simulink model "StandardModel_tl"  (Simulink 7.5)
settings: Solver=FixedStepDiscrete  StartTime=0.0  StopTime=10.0  FixedStep=0.01  RelTol=1e-3
PreLoadFcn:
  | if exist('tl_preloadfcn','file'), tl_preloadfcn(gcs,101); end
PostLoadFcn:
  | if exist('tl_postloadfcn','file'), tl_postloadfcn(gcs,101); end
InitFcn:
  | if exist('tlds_init','file'), tlds_init(gcs); end
StartFcn:
  | if exist('tlds_start','file'), tlds_start(gcs); end
StopFcn:
  | if exist('tlds_stop','file'), tlds_stop(gcs); end
libraries: tllib x6
PreSaveFcn:
  | if exist('tl_presavefcn','file'), tl_presavefcn(gcs); end
settings Model: DS_PROJECTFILE=StandardModel.dd  TL_MAIN_DATA={'codeopt',{'optlevel',0,'stateactcodinglimit',1},'logopt',{'plotinterval',0.1},'date',735991.67578921292,'advcodeopt',{'ExtendedBlockComments';'on';'GenerateEmptyConditionalBranches';'on';'PolySpaceSupport';'on'}}  TLRevision=101  Creator=alex  LastModifiedBy=alex  BufferReuse=off
settings DataIOCC: SaveFormat=StructureWithTime
settings OptimizationCC: BlockReduction=off  OptimizeBlockIOStorage=off  BufferReuse=off  ExpressionFolding=off  LocalBlockOutputs=off  InitFltsAndDblsToZero=on
settings DebuggingCC: SaveWithParameterizedLinksMsg=none  SignalResolutionControl=TryResolveAllWithWarning  MultiTaskDSMMsg=warning  MultiTaskCondExecSysMsg=none
settings RTWCC: IncludeERTFirstTime=on
settings GRTTargetCC: TargetFcnLib=ansi_tfl_tmw.mat

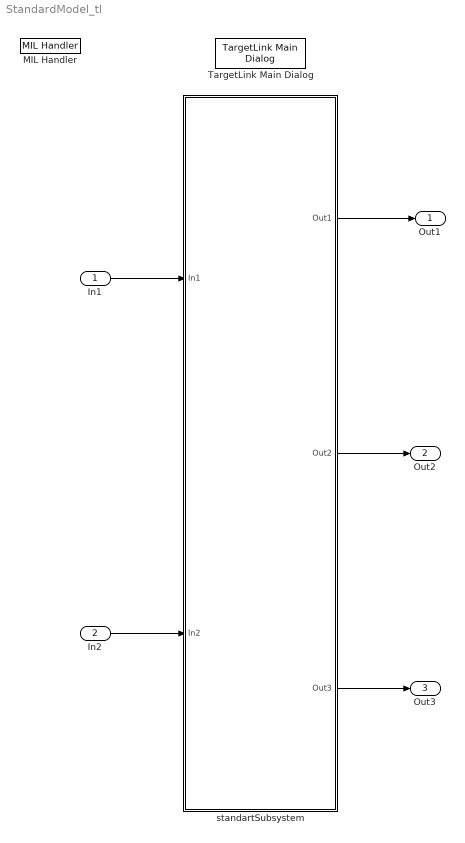
== system StandardModel_tl ==
  In1 : Inport  OutDataType=sfix(16)  OutScaling=2^0
  In2 : Inport  Port=2  OutDataType=sfix(16)  OutScaling=2^0
  MIL Handler : tllib/MIL Handler  data={'date',735991.67578725691}
  TargetLink Main Dialog : tllib/TargetLink Main Dialog  SystemSampleTime=-1
  standartSubsystem : Subsystem  Tag=TargetLink Simulation Frame
      settings: CopyFcn=if exist('tl_copyfcn','file'), tl_copyfcn(gcbh); end  NameChangeFcn=if exist('tl_framenamechangefcn','file'), tl_framenamechangefcn(gcbh); end
      settings: OpenFcn=|
      | if exist('open_tlsubsystem','file')
      |    open_tlsubsystem(gcbh);
      | else
      |    tlsubsystem = ...
      |       find_system(gcb, ...
      |       'LookUnderMasks','on', ...
      |       'FollowLinks','on', ...
      |       'Tag','MIL Subsystem');
      |    open_system(tlsubsystem);
      | end
      mask Type: TL_SimFrame
      mask Display: disp('TargetLink\nModel-\nin-the-loop\nmode')
  Out1 : Outport  OutDataType=sfix(16)  OutScaling=2^0
  Out2 : Outport  Port=2  OutDataType=sfix(16)  OutScaling=2^0
  Out3 : Outport  Port=3  OutDataType=sfix(16)  OutScaling=2^0
  wires:
  In1/1 -> standartSubsystem/1(In1)
  In2/1 -> standartSubsystem/2(In2)
  standartSubsystem/1(Out1) -> Out1/1
  standartSubsystem/2(Out2) -> Out2/1
  standartSubsystem/3(Out3) -> Out3/1

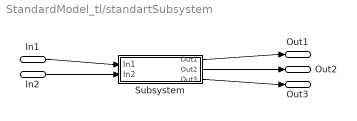
== system StandardModel_tl/standartSubsystem ==
  In1 : Inport  OutDataType=sfix(16)  OutScaling=2^0
  In2 : Inport  Port=2  OutDataType=sfix(16)  OutScaling=2^0
  Subsystem : Subsystem
      settings: OpenFcn=warndlg(get_param(gcb,'MaskHelp'),'Serious Warning');
      mask Type: TL_Enable
      mask Help: This subsystem keeps the TargetLink subsystem (subsystem with TargetLink blocks for production code generation), and is needed for the TargetLink simulation frame to work properly. DO NOT DELETE OR MODIFY IT!
  Out1 : Outport  OutDataType=sfix(16)  OutScaling=2^0
  Out2 : Outport  Port=2  OutDataType=sfix(16)  OutScaling=2^0
  Out3 : Outport  Port=3  OutDataType=sfix(16)  OutScaling=2^0
  wires:
  In1/1 -> Subsystem/1(In1)
  In2/1 -> Subsystem/2(In2)
  Subsystem/1(Out1) -> Out1/1
  Subsystem/2(Out2) -> Out2/1
  Subsystem/3(Out3) -> Out3/1

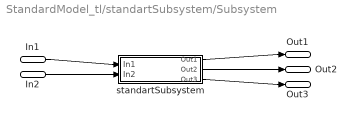
== system StandardModel_tl/standartSubsystem/Subsystem ==
  In1 : Inport  OutDataType=sfix(16)  OutScaling=2^0
  In2 : Inport  Port=2  OutDataType=sfix(16)  OutScaling=2^0
  standartSubsystem : Subsystem  Tag=MIL Subsystem  Description=a
      settings: CopyFcn=if exist('tl_copyfcn','file'), tl_copyfcn(gcbh); end  NameChangeFcn=if exist('tl_namechangefcn','file'), tl_namechangefcn(gcbh); end  DestroyFcn=if exist('update_tl_main_dlg','file'), update_tl_main_dlg('TL_subs_display'); end
      mask Display: disp('TargetLink Subsystem')
  Out1 : Outport  OutDataType=sfix(16)  OutScaling=2^0
  Out2 : Outport  Port=2  OutDataType=sfix(16)  OutScaling=2^0
  Out3 : Outport  Port=3  OutDataType=sfix(16)  OutScaling=2^0
  wires:
  In1/1 -> standartSubsystem/1(In1)
  In2/1 -> standartSubsystem/2(In2)
  standartSubsystem/1(Out1) -> Out1/1
  standartSubsystem/2(Out2) -> Out2/1
  standartSubsystem/3(Out3) -> Out3/1

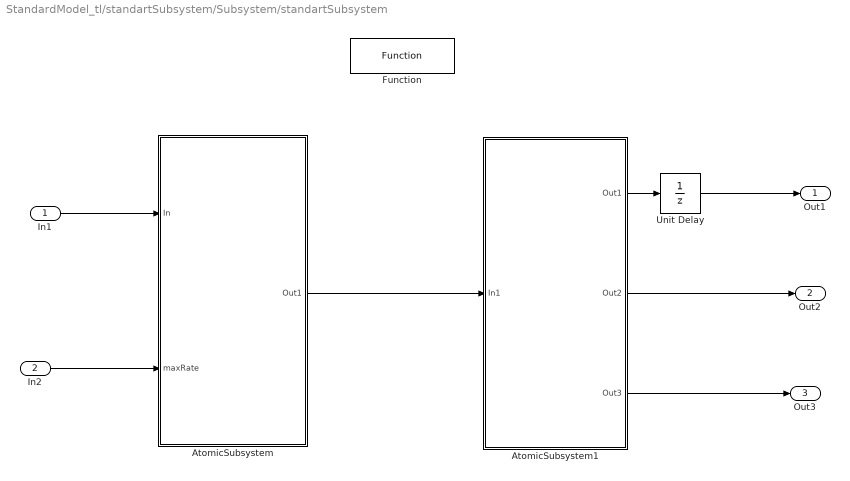
== system StandardModel_tl/standartSubsystem/Subsystem/standartSubsystem ==
  In1 : Inport  PortDimensions=1  OutDataType=sfix(16)  OutScaling=2^0  mask(TL_Inport){data={'logdata',{'plotchannels',[]},'date',735991.6757871412}}
      settings: DeleteFcn=if exist('delete_tlblock','file')==2,delete_tlblock(gcbh);end  OpenFcn=if exist('tl_open_blockdlg','file')==2,tl_open_blockdlg(gcbh);else,open_system(gcbh,'parameter');end
      settings: CopyFcn=|
      | if exist('tl_reset_reviewflag','file')==2
      |     tl_reset_reviewflag(gcbh);
      | end
      | if exist('tl_check_ports','file')
      |     tl_check_ports(gcbh);
      | end
      settings: NameChangeFcn=|
      | if exist('rename_tlblock','file')==2,rename_tlblock(gcbh);end
      | if exist('tl_check_ports','file'), tl_check_ports(gcbh); end
      mask Help: eval(['if exist(''tl_online_help'',''file'') == 2, tl_online_help(''Topic'',''TL_Inport''),else, web([''jar:file:///'',matlabroot,''/help/toolbox/simulink/help.jar!/slref/' lower(get_param(gcbh,'Blocktype')) '.html''], ''-helpbrowser''),end'])
      mask Display: plot([0.2 0.35 NaN 0.65 0.8],[0 1 NaN 0 1]);
  In2 : Inport  Port=2  PortDimensions=1  OutDataType=sfix(16)  OutScaling=2^0  mask(TL_Inport){data={'logdata',{'plotchannels',[]},'output',{'max',300,'min',-800,'lsb',2^-2,'offset',-4},'date',735991.67578673607}}
      settings: DeleteFcn=if exist('delete_tlblock','file')==2,delete_tlblock(gcbh);end  OpenFcn=if exist('tl_open_blockdlg','file')==2,tl_open_blockdlg(gcbh);else,open_system(gcbh,'parameter');end
      settings: CopyFcn=|
      | if exist('tl_reset_reviewflag','file')==2
      |     tl_reset_reviewflag(gcbh);
      | end
      | if exist('tl_check_ports','file')
      |     tl_check_ports(gcbh);
      | end
      settings: NameChangeFcn=|
      | if exist('rename_tlblock','file')==2,rename_tlblock(gcbh);end
      | if exist('tl_check_ports','file'), tl_check_ports(gcbh); end
      mask Help: eval(['if exist(''tl_online_help'',''file'') == 2, tl_online_help(''Topic'',''TL_Inport''),else, web([''jar:file:///'',matlabroot,''/help/toolbox/simulink/help.jar!/slref/' lower(get_param(gcbh,'Blocktype')) '.html''], ''-helpbrowser''),end'])
      mask Display: plot([0.2 0.35 NaN 0.65 0.8],[0 1 NaN 0 1]);
  AtomicSubsystem : Subsystem  TreatAsAtomicUnit=on
  AtomicSubsystem1 : Subsystem  TreatAsAtomicUnit=on
  Function : tllib/Function  SystemSampleTime=-1  data={'date',735991.67578028934}
  Unit Delay : UnitDelay  X0=-2  SampleTime=-1  mask(TL_UnitDelay){data={'logdata',{'plotchannels',[]},'date',735991.6757827315}}
      settings: CopyFcn=set_param(gcb,'ReferenceBlock',''); set_param(gcb,'Tag','COPIED_DURING_UPGRADE');set_param(gcb,'CopyFcn','');  DeleteFcn=if exist('delete_tlblock','file')==2,delete_tlblock(gcbh);end  NameChangeFcn=if exist('rename_tlblock','file')==2,rename_tlblock(gcbh);end  OpenFcn=if exist('tl_open_blockdlg','file')==2,tl_open_blockdlg(gcbh);else,open_system(gcbh,'parameter');end
      mask Help: eval(['if exist(''tl_online_help'',''file'') == 2, tl_online_help(''Topic'',''TL_UnitDelay''),else, web([''jar:file:///'',matlabroot,''/help/toolbox/simulink/help.jar!/slref/' lower(get_param(gcbh,'Blocktype')) '.html''], ''-helpbrowser''),end'])
      mask Display: plot([-0.05, 1.05, NaN, -0.05, 1.05],[.01, .01, NaN, .99, .99])
  Out1 : Outport  PortDimensions=1  OutDataType=sfix(16)  OutScaling=2^0  mask(TL_Outport){data={'logdata',{'plotchannels',[]},'output',{'lsb',2^-1,'offset',-3,'checkmin',1,'checkmax',1},'date',735991.6757824074}}
      settings: DeleteFcn=if exist('delete_tlblock','file')==2,delete_tlblock(gcbh);end  OpenFcn=if exist('tl_open_blockdlg','file')==2,tl_open_blockdlg(gcbh);else,open_system(gcbh,'parameter');end
      settings: CopyFcn=|
      | if exist('tl_reset_reviewflag','file')==2
      |     tl_reset_reviewflag(gcbh);
      | end
      | if exist('tl_check_ports','file')
      |     tl_check_ports(gcbh);
      | end
      settings: NameChangeFcn=|
      | if exist('rename_tlblock','file')==2,rename_tlblock(gcbh);end
      | if exist('tl_check_ports','file'), tl_check_ports(gcbh); end
      mask Help: eval(['if exist(''tl_online_help'',''file'') == 2, tl_online_help(''Topic'',''TL_Outport''),else, web([''jar:file:///'',matlabroot,''/help/toolbox/simulink/help.jar!/slref/' lower(get_param(gcbh,'Blocktype')) '.html''], ''-helpbrowser''),end'])
      mask Display: plot([0.2 0.35 NaN 0.65 0.8],[0 1 NaN 0 1]);
  Out2 : Outport  Port=2  PortDimensions=1  OutDataType=sfix(16)  OutScaling=2^0  mask(TL_Outport){data={'logdata',{'plotchannels',[]},'date',735991.67578196758}}
      settings: DeleteFcn=if exist('delete_tlblock','file')==2,delete_tlblock(gcbh);end  OpenFcn=if exist('tl_open_blockdlg','file')==2,tl_open_blockdlg(gcbh);else,open_system(gcbh,'parameter');end
      settings: CopyFcn=|
      | if exist('tl_reset_reviewflag','file')==2
      |     tl_reset_reviewflag(gcbh);
      | end
      | if exist('tl_check_ports','file')
      |     tl_check_ports(gcbh);
      | end
      settings: NameChangeFcn=|
      | if exist('rename_tlblock','file')==2,rename_tlblock(gcbh);end
      | if exist('tl_check_ports','file'), tl_check_ports(gcbh); end
      mask Help: eval(['if exist(''tl_online_help'',''file'') == 2, tl_online_help(''Topic'',''TL_Outport''),else, web([''jar:file:///'',matlabroot,''/help/toolbox/simulink/help.jar!/slref/' lower(get_param(gcbh,'Blocktype')) '.html''], ''-helpbrowser''),end'])
      mask Display: plot([0.2 0.35 NaN 0.65 0.8],[0 1 NaN 0 1]);
  Out3 : Outport  Port=3  PortDimensions=1  OutDataType=sfix(16)  OutScaling=2^0  mask(TL_Outport){data={'logdata',{'plotchannels',[]},'output',{'type','Int32'},'date',735991.67578146991}}
      settings: DeleteFcn=if exist('delete_tlblock','file')==2,delete_tlblock(gcbh);end  OpenFcn=if exist('tl_open_blockdlg','file')==2,tl_open_blockdlg(gcbh);else,open_system(gcbh,'parameter');end
      settings: CopyFcn=|
      | if exist('tl_reset_reviewflag','file')==2
      |     tl_reset_reviewflag(gcbh);
      | end
      | if exist('tl_check_ports','file')
      |     tl_check_ports(gcbh);
      | end
      settings: NameChangeFcn=|
      | if exist('rename_tlblock','file')==2,rename_tlblock(gcbh);end
      | if exist('tl_check_ports','file'), tl_check_ports(gcbh); end
      mask Help: eval(['if exist(''tl_online_help'',''file'') == 2, tl_online_help(''Topic'',''TL_Outport''),else, web([''jar:file:///'',matlabroot,''/help/toolbox/simulink/help.jar!/slref/' lower(get_param(gcbh,'Blocktype')) '.html''], ''-helpbrowser''),end'])
      mask Display: plot([0.2 0.35 NaN 0.65 0.8],[0 1 NaN 0 1]);
  wires:
  AtomicSubsystem1/3(Out3) -> Out3/1
  AtomicSubsystem1/2(Out2) -> Out2/1
  Unit Delay/1 -> Out1/1
  In2/1 -> AtomicSubsystem/2(maxRate)
  In1/1 -> AtomicSubsystem/1(In)
  AtomicSubsystem/1(Out1) -> AtomicSubsystem1/1(In1)
  AtomicSubsystem1/1(Out1) -> Unit Delay/1

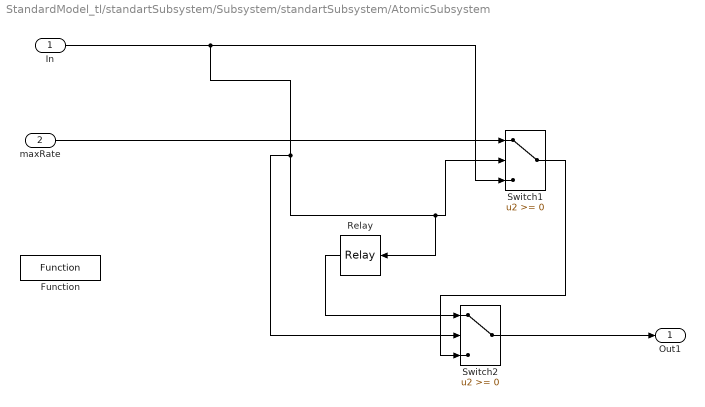
== system StandardModel_tl/standartSubsystem/Subsystem/standartSubsystem/AtomicSubsystem ==
  In : Inport  PortDimensions=1  OutDataType=sfix(16)  OutScaling=2^0  mask(TL_Inport){data={'logdata',{'plotchannels',[]},'output',{'class','FCN_ARG'},'date',735991.67578631942}}
      settings: CopyFcn=if exist('tl_reset_reviewflag','file')==2,tl_reset_reviewflag(gcbh);end  DeleteFcn=if exist('delete_tlblock','file')==2,delete_tlblock(gcbh);end  NameChangeFcn=if exist('rename_tlblock','file')==2,rename_tlblock(gcbh);end  OpenFcn=if exist('tl_open_blockdlg','file')==2,tl_open_blockdlg(gcbh);else,open_system(gcbh,'parameter');end
      mask Help: eval(['if exist(''tl_online_help'',''file'') == 2, tl_online_help(''Topic'',''TL_Inport''),else, web([''jar:file:///'',matlabroot,''/help/toolbox/simulink/help.jar!/slref/' lower(get_param(gcbh,'Blocktype')) '.html''], ''-helpbrowser''),end'])
      mask Display: plot([0.2 0.35 NaN 0.65 0.8],[0 1 NaN 0 1]);
  maxRate : Inport  Port=2  PortDimensions=1  OutDataType=sfix(16)  OutScaling=2^0  mask(TL_Inport){data={'logdata',{'plotchannels',[]},'output',{'class','FCN_REF_ARG'},'date',735991.6757859143}}
      settings: CopyFcn=if exist('tl_reset_reviewflag','file')==2,tl_reset_reviewflag(gcbh);end  DeleteFcn=if exist('delete_tlblock','file')==2,delete_tlblock(gcbh);end  NameChangeFcn=if exist('rename_tlblock','file')==2,rename_tlblock(gcbh);end  OpenFcn=if exist('tl_open_blockdlg','file')==2,tl_open_blockdlg(gcbh);else,open_system(gcbh,'parameter');end
      mask Help: eval(['if exist(''tl_online_help'',''file'') == 2, tl_online_help(''Topic'',''TL_Inport''),else, web([''jar:file:///'',matlabroot,''/help/toolbox/simulink/help.jar!/slref/' lower(get_param(gcbh,'Blocktype')) '.html''], ''-helpbrowser''),end'])
      mask Display: plot([0.2 0.35 NaN 0.65 0.8],[0 1 NaN 0 1]);
  Function : tllib/Function  SystemSampleTime=-1  data={'stepfunctionclass','STATIC_FCN','date',735991.6757809954}
  Relay : Relay  OnSwitchValue=1  OffSwitchValue=-1  OutDataType=sfix(16)  OutScaling=2^0  mask(TL_Relay){data={'logdata',{'plotchannels',[]},'onoutput',{'class','CAL'},'offoutput',{'class','CAL'},'onswitch',{'class','CAL'},'offswitch',{'class','CAL'},'date',735991.67578543979}}
      settings: CopyFcn=set_param(gcb,'ReferenceBlock',''); set_param(gcb,'Tag','COPIED_DURING_UPGRADE');set_param(gcb,'CopyFcn','');  DeleteFcn=if exist('delete_tlblock','file')==2,delete_tlblock(gcbh);end  NameChangeFcn=if exist('rename_tlblock','file')==2,rename_tlblock(gcbh);end  OpenFcn=if exist('tl_open_blockdlg','file')==2,tl_open_blockdlg(gcbh);else,open_system(gcbh,'parameter');end
      mask Help: eval(['if exist(''tl_online_help'',''file'') == 2, tl_online_help(''Topic'',''TL_Relay''),else, web([''jar:file:///'',matlabroot,''/help/toolbox/simulink/help.jar!/slref/' lower(get_param(gcbh,'Blocktype')) '.html''], ''-helpbrowser''),end'])
      mask Display: plot([-0.05, 1.05, NaN, -0.05, 1.05],[.01, .01, NaN, .99, .99])
  Switch1 : Switch  OutDataType=sfix(16)  OutScaling=2^0  SaturateOnIntegerOverflow=on  InputSameDT=on  mask(TL_Switch){data={'logdata',{'plotchannels',[]},'threshold',{'class','CAL'},'date',735991.67578491895}}
      settings: CopyFcn=set_param(gcb,'ReferenceBlock',''); set_param(gcb,'Tag','COPIED_DURING_UPGRADE');set_param(gcb,'CopyFcn','');  DeleteFcn=if exist('delete_tlblock','file')==2,delete_tlblock(gcbh);end  NameChangeFcn=if exist('rename_tlblock','file')==2,rename_tlblock(gcbh);end  OpenFcn=if exist('tl_open_blockdlg','file')==2,tl_open_blockdlg(gcbh);else,open_system(gcbh,'parameter');end
      mask Help: eval(['if exist(''tl_online_help'',''file'') == 2, tl_online_help(''Topic'',''TL_Switch''),else, web([''jar:file:///'',matlabroot,''/help/toolbox/simulink/help.jar!/slref/' lower(get_param(gcbh,'Blocktype')) '.html''], ''-helpbrowser''),end'])
      mask Display: plot([-0.05, 1.05, NaN, -0.05, 1.05],[.01, .01, NaN, .99, .99])
  Switch2 : Switch  OutDataType=sfix(16)  OutScaling=2^0  SaturateOnIntegerOverflow=on  InputSameDT=on  mask(TL_Switch){data={'logdata',{'plotchannels',[]},'threshold',{'class','CAL'},'date',735991.67578460649}}
      settings: CopyFcn=set_param(gcb,'ReferenceBlock',''); set_param(gcb,'Tag','COPIED_DURING_UPGRADE');set_param(gcb,'CopyFcn','');  DeleteFcn=if exist('delete_tlblock','file')==2,delete_tlblock(gcbh);end  NameChangeFcn=if exist('rename_tlblock','file')==2,rename_tlblock(gcbh);end  OpenFcn=if exist('tl_open_blockdlg','file')==2,tl_open_blockdlg(gcbh);else,open_system(gcbh,'parameter');end
      mask Help: eval(['if exist(''tl_online_help'',''file'') == 2, tl_online_help(''Topic'',''TL_Switch''),else, web([''jar:file:///'',matlabroot,''/help/toolbox/simulink/help.jar!/slref/' lower(get_param(gcbh,'Blocktype')) '.html''], ''-helpbrowser''),end'])
      mask Display: plot([-0.05, 1.05, NaN, -0.05, 1.05],[.01, .01, NaN, .99, .99])
  Out1 : Outport  PortDimensions=1  OutDataType=sfix(16)  OutScaling=2^0  mask(TL_Outport){data={'logdata',{'plotchannels',[]},'output',{'class','FCN_RETURN'},'date',735991.67578423605}}
      settings: CopyFcn=if exist('tl_reset_reviewflag','file')==2,tl_reset_reviewflag(gcbh);end  DeleteFcn=if exist('delete_tlblock','file')==2,delete_tlblock(gcbh);end  NameChangeFcn=if exist('rename_tlblock','file')==2,rename_tlblock(gcbh);end  OpenFcn=if exist('tl_open_blockdlg','file')==2,tl_open_blockdlg(gcbh);else,open_system(gcbh,'parameter');end
      mask Help: eval(['if exist(''tl_online_help'',''file'') == 2, tl_online_help(''Topic'',''TL_Outport''),else, web([''jar:file:///'',matlabroot,''/help/toolbox/simulink/help.jar!/slref/' lower(get_param(gcbh,'Blocktype')) '.html''], ''-helpbrowser''),end'])
      mask Display: plot([0.2 0.35 NaN 0.65 0.8],[0 1 NaN 0 1]);
  wires:
  Relay/1 -> Switch2/1
  Switch1/1 -> Switch2/3
  Switch2/1 -> Out1/1
  maxRate/1 -> Switch1/1
  In/1 -> Switch1/3, Switch1/2, Relay/1, Switch2/2

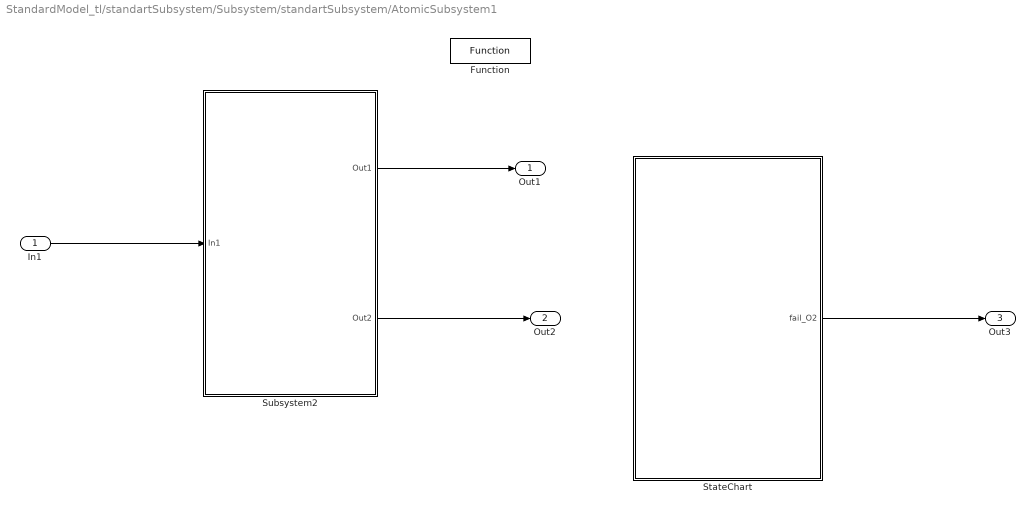
== system StandardModel_tl/standartSubsystem/Subsystem/standartSubsystem/AtomicSubsystem1 ==
  In1 : Inport  OutDataType=sfix(16)  OutScaling=2^0
  Function : tllib/Function  SystemSampleTime=-1  data={'date',735991.67578077549}
  StateChart : Stateflow chart  Description=Stateflow diagram to determine control system operating mode  TreatAsAtomicUnit=on
  Subsystem2 : Subsystem  TreatAsAtomicUnit=on
  Out1 : Outport  OutDataType=sfix(16)  OutScaling=2^0
  Out2 : Outport  Port=2  OutDataType=sfix(16)  OutScaling=2^0
  Out3 : Outport  Port=3  OutDataType=sfix(16)  OutScaling=2^0
  wires:
  Subsystem2/2(Out2) -> Out2/1
  In1/1 -> Subsystem2/1(In1)
  Subsystem2/1(Out1) -> Out1/1
  StateChart/1(fail_O2) -> Out3/1

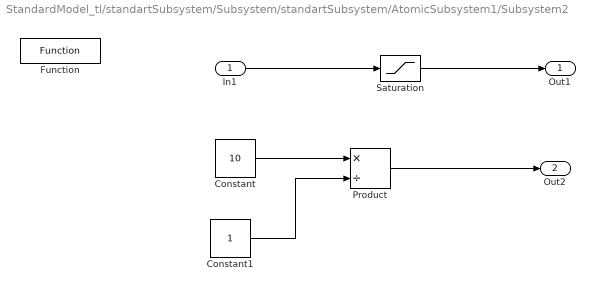
== system StandardModel_tl/standartSubsystem/Subsystem/standartSubsystem/AtomicSubsystem1/Subsystem2 ==
  In1 : Inport  OutDataType=sfix(16)  OutScaling=2^0
  Constant : Constant  Value=10  OutDataType=sfix(16)  OutScaling=2^0  mask(TL_Constant){data={'output',{'class','GLOBAL'},'date',735991.6757838194}}
      settings: CopyFcn=set_param(gcb,'ReferenceBlock',''); set_param(gcb,'Tag','COPIED_DURING_UPGRADE');set_param(gcb,'CopyFcn','');  DeleteFcn=if exist('delete_tlblock','file')==2,delete_tlblock(gcbh);end  NameChangeFcn=if exist('rename_tlblock','file')==2,rename_tlblock(gcbh);end  OpenFcn=if exist('tl_open_blockdlg','file')==2,tl_open_blockdlg(gcbh);else,open_system(gcbh,'parameter');end
      mask Help: eval(['if exist(''tl_online_help'',''file'') == 2, tl_online_help(''Topic'',''TL_Constant''),else, web([''jar:file:///'',matlabroot,''/help/toolbox/simulink/help.jar!/slref/' lower(get_param(gcbh,'Blocktype')) '.html''], ''-helpbrowser''),end'])
      mask Display: plot([-0.05, 1.05, NaN, -0.05, 1.05],[.01, .01, NaN, .99, .99])
  Constant1 : Constant  OutDataType=sfix(16)  OutScaling=2^0  mask(TL_Constant){data={'output',{'class','CAL'},'date',735991.67578361114}}
      settings: CopyFcn=set_param(gcb,'ReferenceBlock',''); set_param(gcb,'Tag','COPIED_DURING_UPGRADE');set_param(gcb,'CopyFcn','');  DeleteFcn=if exist('delete_tlblock','file')==2,delete_tlblock(gcbh);end  NameChangeFcn=if exist('rename_tlblock','file')==2,rename_tlblock(gcbh);end  OpenFcn=if exist('tl_open_blockdlg','file')==2,tl_open_blockdlg(gcbh);else,open_system(gcbh,'parameter');end
      mask Help: eval(['if exist(''tl_online_help'',''file'') == 2, tl_online_help(''Topic'',''TL_Constant''),else, web([''jar:file:///'',matlabroot,''/help/toolbox/simulink/help.jar!/slref/' lower(get_param(gcbh,'Blocktype')) '.html''], ''-helpbrowser''),end'])
      mask Display: plot([-0.05, 1.05, NaN, -0.05, 1.05],[.01, .01, NaN, .99, .99])
  Function : tllib/Function  SystemSampleTime=-1  data={'date',735991.67578054394}
  Product : Product  Inputs=*/  OutDataType=sfix(16)  OutScaling=2^0  RndMeth=Zero  mask(TL_Product){data={'logdata',{'plotchannels',[]},'date',735991.67578336806}}
      settings: CopyFcn=set_param(gcb,'ReferenceBlock',''); set_param(gcb,'Tag','COPIED_DURING_UPGRADE');set_param(gcb,'CopyFcn','');  DeleteFcn=if exist('delete_tlblock','file')==2,delete_tlblock(gcbh);end  NameChangeFcn=if exist('rename_tlblock','file')==2,rename_tlblock(gcbh);end  OpenFcn=if exist('tl_open_blockdlg','file')==2,tl_open_blockdlg(gcbh);else,open_system(gcbh,'parameter');end
      mask Help: eval(['if exist(''tl_online_help'',''file'') == 2, tl_online_help(''Topic'',''TL_Product''),else, web([''jar:file:///'',matlabroot,''/help/toolbox/simulink/help.jar!/slref/' lower(get_param(gcbh,'Blocktype')) '.html''], ''-helpbrowser''),end'])
      mask Display: plot([-0.05, 1.05, NaN, -0.05, 1.05],[.01, .01, NaN, .99, .99])
  Saturation : Saturate  UpperLimit=2  LowerLimit=0  OutDataType=sfix(16)  OutScaling=2^0  mask(TL_Saturate){data={'logdata',{'plotchannels',[]},'output',{'max',255,'min',0,'type','uint16'},'lowerlimit',{'class','CAL'},'upperlimit',{'class','CAL'},'date',735991.67578311346}}
      settings: CopyFcn=set_param(gcb,'ReferenceBlock',''); set_param(gcb,'Tag','COPIED_DURING_UPGRADE');set_param(gcb,'CopyFcn','');  DeleteFcn=if exist('delete_tlblock','file')==2,delete_tlblock(gcbh);end  NameChangeFcn=if exist('rename_tlblock','file')==2,rename_tlblock(gcbh);end  OpenFcn=if exist('tl_open_blockdlg','file')==2,tl_open_blockdlg(gcbh);else,open_system(gcbh,'parameter');end
      mask Help: eval(['if exist(''tl_online_help'',''file'') == 2, tl_online_help(''Topic'',''TL_Saturate''),else, web([''jar:file:///'',matlabroot,''/help/toolbox/simulink/help.jar!/slref/' lower(get_param(gcbh,'Blocktype')) '.html''], ''-helpbrowser''),end'])
      mask Display: plot([-0.05, 1.05, NaN, -0.05, 1.05],[.01, .01, NaN, .99, .99])
  Out1 : Outport  OutDataType=sfix(16)  OutScaling=2^0
  Out2 : Outport  Port=2  OutDataType=sfix(16)  OutScaling=2^0
  wires:
  In1/1 -> Saturation/1
  Saturation/1 -> Out1/1
  Constant1/1 -> Product/2
  Constant/1 -> Product/1
  Product/1 -> Out2/1

== stateflow chart standartSubsystem/Subsystem/standartSubsystem/AtomicSubsystem1/StateChart ==
  settings: updateMethod=DISCRETE  sampleTime=0.01  description=$TL$ functionname=$O; $TL$
  state OxygenSensMode [parallel]
    settings: executionOrder=1
    settings: description=|
        | This state determines the validity of the exhaust gas oxygen sensor (EGO) data.
        | $TL$ name=$C_X_$O$R; $TL$
    state O2_Normal
      entry: fail_O2 = 0;
      settings: description=|
          | Normal EGO sensor operation gives a reliable indication of excess oxygen in the exhaust gas, from which air/fuel mixture can be inferred.
          | $TL$ name=$C_X_$O$R; $TL$
    state O2_Fail
      entry: fail_O2 = 1;
      settings: description=|
          | The EGO sensor has failed.
          | $TL$ name=$C_X_$O$R; $TL$
    state O2_Warmup
      entry: fail_O2 = 1;
      settings: description=|
          | The EGO sensor must come up to temperature before its data is reliable.
          | $TL$ name=$C_X_$O$R; $TL$
    O2_Warmup -> O2_Normal : [Calvariable== 5]
      settings: description=It is assumed that the time o2_t_thresh is sufficient for the sensor to warm up to operational temperature.
    (default) -> O2_Warmup
    O2_Normal -> O2_Fail : [Calvariable == 7]
      settings: description=The failure condition is indicated by excessive output voltage.
  data: Calvariable parameter int32 [0..1] =1; fail_O2 output int32 [0..1]
  data Calvariable settings: description=|
      | minimum manifold pressure expected at zero speed
      | $TL$ name=$C_V_$O$R; type=Int32; class=CAL; $TL$
  data fail_O2 settings: description=|
      | failure of oxygene sensor
      | $TL$ name=$O; type=Int32; class=MERGEABLE_DISP; $TL$
